simulink model "CurrentRegulationandFeedbackComponent"  (R2026a)
settings: Solver=FixedStepDiscrete
settings Model: DataDictionary=TractionEmotorSoftwareArchInterfaceData.sldd  Creator=dakaihu  LastModifiedBy=dakaihu

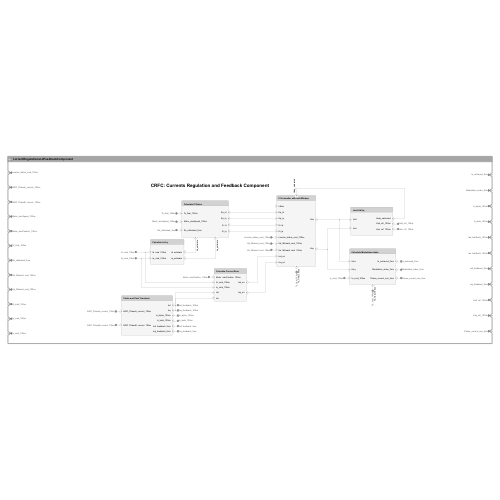
[thumbnail: Simulink's stored preview of the top-level diagram]
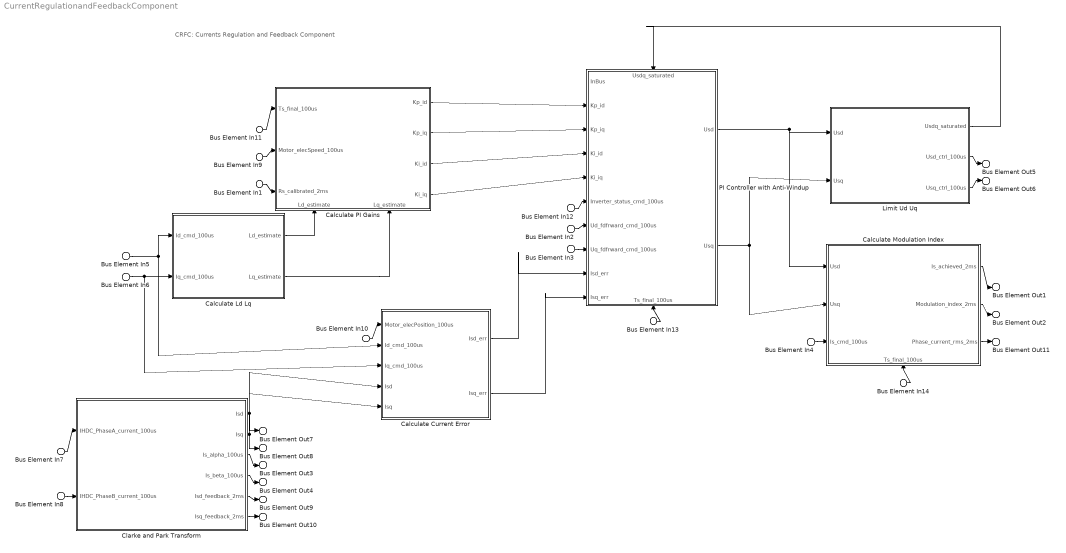
== system CurrentRegulationandFeedbackComponent ==
  note: CRFC: Currents Regulation and Feedback Component
  Bus Element In12 : Inport  PortName=Inverter_status_cmd_100us
  Bus Element In7 : Inport  Port=2  PortName=IHDC_PhaseA_current_100us
  Bus Element In8 : Inport  Port=3  PortName=IHDC_PhaseB_current_100us
  Bus Element In9 : Inport  Port=4  PortName=Motor_elecSpeed_100us
  Bus Element In10 : Inport  Port=5  PortName=Motor_elecPosition_100us
  Bus Element In11 : Inport  Port=6  PortName=Ts_final_100us
  Bus Element In13 : Inport  Port=6  PortName=Ts_final_100us
  Bus Element In14 : Inport  Port=6  PortName=Ts_final_100us
  Bus Element In1 : Inport  Port=7  PortName=Rs_calibrated_2ms
  Bus Element In2 : Inport  Port=8  PortName=Ud_fdfrward_cmd_100us
  Bus Element In3 : Inport  Port=9  PortName=Uq_fdfrward_cmd_100us
  Bus Element In5 : Inport  Port=10  PortName=Id_cmd_100us
  Bus Element In6 : Inport  Port=11  PortName=Iq_cmd_100us
  Bus Element In4 : Inport  Port=12  PortName=Is_cmd_100us
  "Calculate Current Error " : Subsystem
      settings: PortSchema="{\"entries\":[{\"content\":{\"headerSize\":26,\"margin\":15,\"minimumSpacing\":25,\"sides\":[{\"content\":{\"connectorIds\":[\"In1\",\"In2\",\"In3\",\"In4\",\"In5\"]},\"type\":\"ConnectorPlacement.EquallySpacedRectSide\",\"uuid\":\"48197cfa-225d-469b-bade-a4603c3ad603\"},{\"content\":{\"connectorIds\":[\"Out1\",\"Out2\"],\"side\":\"RIGHT\"},\"type\":\"ConnectorPlacement.EquallySpacedRectSide\",\"uuid\":\"66f990f6-adbc-4e6f-80ea-1c4f0b5a4b64\"},{\"content\":{\"connectorIds\":[],\"side\":\"TOP\"},\"type\":\"ConnectorPlacement.EquallySpacedRectSide\",\"uuid\":\"942001c3-a853-4b04-81e7-4a7a1fb8bb28\"}]},\"type\":\"ConnectorPlacement.EquallySpacedConnector\",\"uuid\":\"eed822cb-7078-4505-8d8e-0c793411ce34\"}],\"packageUris\":[\"http://schema.mathworks.com/mf0/Connector/R2020b\"],\"version\":\"1.0\"}"
  Calculate Ld Lq : Subsystem
      settings: PortSchema="{\"entries\":[{\"content\":{\"headerSize\":26,\"margin\":15,\"minimumSpacing\":25,\"sides\":[{\"content\":{\"connectorIds\":[\"In1\",\"In2\"]},\"type\":\"ConnectorPlacement.EquallySpacedRectSide\",\"uuid\":\"48197cfa-225d-469b-bade-a4603c3ad603\"},{\"content\":{\"connectorIds\":[\"Out1\",\"Out2\"],\"side\":\"RIGHT\"},\"type\":\"ConnectorPlacement.EquallySpacedRectSide\",\"uuid\":\"66f990f6-adbc-4e6f-80ea-1c4f0b5a4b64\"},{\"content\":{\"connectorIds\":[],\"side\":\"TOP\"},\"type\":\"ConnectorPlacement.EquallySpacedRectSide\",\"uuid\":\"942001c3-a853-4b04-81e7-4a7a1fb8bb28\"}]},\"type\":\"ConnectorPlacement.EquallySpacedConnector\",\"uuid\":\"eed822cb-7078-4505-8d8e-0c793411ce34\"}],\"packageUris\":[\"http://schema.mathworks.com/mf0/Connector/R2020b\"],\"version\":\"1.0\"}"
  Calculate Modulation Index : Subsystem
      settings: PortSchema="{\"entries\":[{\"content\":{\"headerSize\":26,\"margin\":15,\"minimumSpacing\":25,\"sides\":[{\"content\":{\"connectorIds\":[\"In2\",\"In3\",\"In4\"]},\"type\":\"ConnectorPlacement.EquallySpacedRectSide\",\"uuid\":\"48197cfa-225d-469b-bade-a4603c3ad603\"},{\"content\":{\"connectorIds\":[\"Out1\",\"Out2\",\"Out3\"],\"side\":\"RIGHT\"},\"type\":\"ConnectorPlacement.EquallySpacedRectSide\",\"uuid\":\"66f990f6-adbc-4e6f-80ea-1c4f0b5a4b64\"},{\"content\":{\"connectorIds\":[],\"side\":\"TOP\"},\"type\":\"ConnectorPlacement.EquallySpacedRectSide\",\"uuid\":\"942001c3-a853-4b04-81e7-4a7a1fb8bb28\"},{\"content\":{\"connectorIds\":[\"In1\"],\"side\":\"BOTTOM\"},\"type\":\"ConnectorPlacement.EquallySpacedRectSide\",\"uuid\":\"b02502b0-0db1-4dfc-a3e2-057df5b912de\"}]},\"type\":\"ConnectorPlacement.EquallySpacedConnector\",\"uuid\":\"eed822cb-7078-4505-8d8e-0c793411ce34\"}],\"packageUris\":[\"http://schema.mathworks.com/mf0/Connector/R2020b\"],\"version\":\"1.0\"}"
  Calculate PI Gains : Subsystem
      settings: PortSchema="{\"entries\":[{\"content\":{\"headerSize\":26,\"margin\":15,\"minimumSpacing\":25,\"sides\":[{\"content\":{\"connectorIds\":[\"In1\",\"In2\",\"In3\"]},\"type\":\"ConnectorPlacement.EquallySpacedRectSide\",\"uuid\":\"48197cfa-225d-469b-bade-a4603c3ad603\"},{\"content\":{\"connectorIds\":[\"Out1\",\"Out2\",\"Out4\",\"Out3\"],\"side\":\"RIGHT\"},\"type\":\"ConnectorPlacement.EquallySpacedRectSide\",\"uuid\":\"66f990f6-adbc-4e6f-80ea-1c4f0b5a4b64\"},{\"content\":{\"connectorIds\":[],\"side\":\"TOP\"},\"type\":\"ConnectorPlacement.EquallySpacedRectSide\",\"uuid\":\"942001c3-a853-4b04-81e7-4a7a1fb8bb28\"},{\"content\":{\"connectorIds\":[\"In4\",\"In5\"],\"side\":\"BOTTOM\"},\"type\":\"ConnectorPlacement.EquallySpacedRectSide\",\"uuid\":\"3d9d326e-8475-49e8-bdf1-4ba0dc1e2f42\"}]},\"type\":\"ConnectorPlacement.EquallySpacedConnector\",\"uuid\":\"eed822cb-7078-4505-8d8e-0c793411ce34\"}],\"packageUris\":[\"http://schema.mathworks.com/mf0/Connector/R2020b\"],\"version\":\"1.0\"}"
  Clarke and Park Transform : Subsystem
      settings: PortSchema="{\"entries\":[{\"content\":{\"headerSize\":26,\"margin\":15,\"minimumSpacing\":25,\"sides\":[{\"content\":{\"connectorIds\":[\"In1\",\"In2\"]},\"type\":\"ConnectorPlacement.EquallySpacedRectSide\",\"uuid\":\"48197cfa-225d-469b-bade-a4603c3ad603\"},{\"content\":{\"connectorIds\":[\"Out1\",\"Out2\",\"Out3\",\"Out4\",\"Out5\",\"Out6\"],\"side\":\"RIGHT\"},\"type\":\"ConnectorPlacement.EquallySpacedRectSide\",\"uuid\":\"66f990f6-adbc-4e6f-80ea-1c4f0b5a4b64\"},{\"content\":{\"connectorIds\":[],\"side\":\"TOP\"},\"type\":\"ConnectorPlacement.EquallySpacedRectSide\",\"uuid\":\"942001c3-a853-4b04-81e7-4a7a1fb8bb28\"}]},\"type\":\"ConnectorPlacement.EquallySpacedConnector\",\"uuid\":\"eed822cb-7078-4505-8d8e-0c793411ce34\"}],\"packageUris\":[\"http://schema.mathworks.com/mf0/Connector/R2020b\"],\"version\":\"1.0\"}"
  Limit Ud Uq : Subsystem
      settings: PortSchema="{\"entries\":[{\"content\":{\"headerSize\":26,\"margin\":15,\"minimumSpacing\":25,\"sides\":[{\"content\":{\"connectorIds\":[\"In1\",\"In2\"]},\"type\":\"ConnectorPlacement.EquallySpacedRectSide\",\"uuid\":\"48197cfa-225d-469b-bade-a4603c3ad603\"},{\"content\":{\"connectorIds\":[\"Out1\",\"Out2\",\"Out3\"],\"side\":\"RIGHT\"},\"type\":\"ConnectorPlacement.EquallySpacedRectSide\",\"uuid\":\"66f990f6-adbc-4e6f-80ea-1c4f0b5a4b64\"},{\"content\":{\"connectorIds\":[],\"side\":\"TOP\"},\"type\":\"ConnectorPlacement.EquallySpacedRectSide\",\"uuid\":\"942001c3-a853-4b04-81e7-4a7a1fb8bb28\"}]},\"type\":\"ConnectorPlacement.EquallySpacedConnector\",\"uuid\":\"eed822cb-7078-4505-8d8e-0c793411ce34\"}],\"packageUris\":[\"http://schema.mathworks.com/mf0/Connector/R2020b\"],\"version\":\"1.0\"}"
  PI Controller with Anti-Windup : Subsystem
      settings: PortSchema="{\"entries\":[{\"content\":{\"headerSize\":26,\"margin\":15,\"minimumSpacing\":25,\"sides\":[{\"content\":{\"connectorIds\":[\"In2\",\"In5\",\"In6\",\"In7\",\"In8\",\"In4\",\"In9\",\"In10\",\"In11\",\"In12\"]},\"type\":\"ConnectorPlacement.EquallySpacedRectSide\",\"uuid\":\"48197cfa-225d-469b-bade-a4603c3ad603\"},{\"content\":{\"connectorIds\":[\"Out1\",\"Out2\"],\"side\":\"RIGHT\"},\"type\":\"ConnectorPlacement.EquallySpacedRectSide\",\"uuid\":\"66f990f6-adbc-4e6f-80ea-1c4f0b5a4b64\"},{\"content\":{\"connectorIds\":[\"In3\"],\"side\":\"TOP\"},\"type\":\"ConnectorPlacement.EquallySpacedRectSide\",\"uuid\":\"942001c3-a853-4b04-81e7-4a7a1fb8bb28\"},{\"content\":{\"connectorIds\":[\"In1\"],\"side\":\"BOTTOM\"},\"type\":\"ConnectorPlacement.EquallySpacedRectSide\",\"uuid\":\"cc117984-18a2-4a20-b6dc-41212c4c98a4\"}]},\"type\":\"ConnectorPlacement.EquallySpacedConnector\",\"uuid\":\"eed822cb-7078-4505-8d8e-0c793411ce34\"}],\"packageUris\":[\"http://schema.mathworks.com/mf0/Connector/R2020b\"],\"version\":\"1.0\"}"
  Bus Element Out1 : Outport  PortName=Is_achieved_2ms
  Bus Element Out2 : Outport  Port=2  PortName=Modulation_index_2ms
  Bus Element Out3 : Outport  Port=3  PortName=Is_alpha_100us
  Bus Element Out4 : Outport  Port=4  PortName=Is_beta_100us
  Bus Element Out7 : Outport  Port=5  PortName=Isd_feedback_100us
  Bus Element Out8 : Outport  Port=6  PortName=Isq_feedback_100us
  Bus Element Out9 : Outport  Port=7  PortName=Isd_feedback_2ms
  Bus Element Out10 : Outport  Port=8  PortName=Isq_feedback_2ms
  Bus Element Out5 : Outport  Port=9  PortName=Usd_ctrl_100us
  Bus Element Out6 : Outport  Port=10  PortName=Usq_ctrl_100us
  Bus Element Out11 : Outport  Port=11  PortName=Phase_current_rms_2ms
  wires:
  Bus Element In5/1 -> "Calculate Current Error "/2(Id_cmd_100us), Calculate Ld Lq/1(Id_cmd_100us)
  Bus Element In6/1 -> "Calculate Current Error "/3(Iq_cmd_100us), Calculate Ld Lq/2(Iq_cmd_100us)
  Calculate Ld Lq/1(Ld_estimate) -> Calculate PI Gains/4(Ld_estimate)
  Calculate Ld Lq/2(Lq_estimate) -> Calculate PI Gains/5(Lq_estimate)
  Bus Element In11/1 -> Calculate PI Gains/1(Ts_final_100us)
  Bus Element In9/1 -> Calculate PI Gains/2(Motor_elecSpeed_100us)
  Bus Element In1/1 -> Calculate PI Gains/3(Rs_calibrated_2ms)
  Calculate PI Gains/1(Kp_id) -> PI Controller with Anti-Windup/5(Kp_id)
  Calculate PI Gains/2(Kp_iq) -> PI Controller with Anti-Windup/6(Kp_iq)
  Calculate PI Gains/4(Ki_id) -> PI Controller with Anti-Windup/7(Ki_id)
  Calculate PI Gains/3(Ki_iq) -> PI Controller with Anti-Windup/8(Ki_iq)
  Bus Element In2/1 -> PI Controller with Anti-Windup/9(Ud_fdfrward_cmd_100us)
  Bus Element In3/1 -> PI Controller with Anti-Windup/10(Uq_fdfrward_cmd_100us)
  Bus Element In12/1 -> PI Controller with Anti-Windup/4(Inverter_status_cmd_100us)
  "Calculate Current Error "/1(Isd_err) -> PI Controller with Anti-Windup/11(Isd_err)
  "Calculate Current Error "/2(Isq_err) -> PI Controller with Anti-Windup/12(Isq_err)
  Bus Element In7/1 -> Clarke and Park Transform/1(IHDC_PhaseA_current_100us)
  Bus Element In8/1 -> Clarke and Park Transform/2(IHDC_PhaseB_current_100us)
  Clarke and Park Transform/3(Is_alpha_100us) -> Bus Element Out3/1
  Clarke and Park Transform/4(Is_beta_100us) -> Bus Element Out4/1
  Bus Element In10/1 -> "Calculate Current Error "/1(Motor_elecPosition_100us)
  PI Controller with Anti-Windup/2(Usq) -> Limit Ud Uq/2(Usq), Calculate Modulation Index/3(Usq)
  Limit Ud Uq/1(Usdq_saturated) -> PI Controller with Anti-Windup/3(Usdq_saturated)
  Bus Element In4/1 -> Calculate Modulation Index/4(Is_cmd_100us)
  Bus Element In13/1 -> PI Controller with Anti-Windup/1(Ts_final_100us)
  Bus Element In14/1 -> Calculate Modulation Index/1(Ts_final_100us)
  Clarke and Park Transform/1(Isd) -> "Calculate Current Error "/4(Isd), Bus Element Out7/1
  Clarke and Park Transform/2(Isq) -> "Calculate Current Error "/5(Isq), Bus Element Out8/1
  Clarke and Park Transform/5(Isd_feedback_2ms) -> Bus Element Out9/1
  Clarke and Park Transform/6(Isq_feedback_2ms) -> Bus Element Out10/1
  Calculate Modulation Index/1(Is_achieved_2ms) -> Bus Element Out1/1
  Calculate Modulation Index/2(Modulation_index_2ms) -> Bus Element Out2/1
  PI Controller with Anti-Windup/1(Usd) -> Limit Ud Uq/1(Usd), Calculate Modulation Index/2(Usd)
  Limit Ud Uq/2(Usd_ctrl_100us) -> Bus Element Out5/1
  Limit Ud Uq/3(Usq_ctrl_100us) -> Bus Element Out6/1
  Calculate Modulation Index/3(Phase_current_rms_2ms) -> Bus Element Out11/1

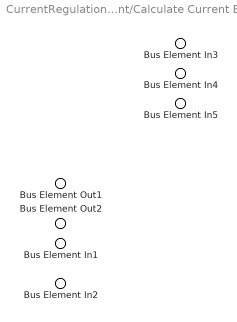
== system CurrentRegulationandFeedbackComponent/Calculate Current Error  ==
  Bus Element In5 : Inport  PortName=Motor_elecPosition_100us
  Bus Element In3 : Inport  Port=2  PortName=Id_cmd_100us
  Bus Element In4 : Inport  Port=3  PortName=Iq_cmd_100us
  Bus Element In1 : Inport  Port=4  PortName=Isd
  Bus Element In2 : Inport  Port=5  PortName=Isq
  Bus Element Out1 : Outport  PortName=Isd_err
  Bus Element Out2 : Outport  Port=2  PortName=Isq_err

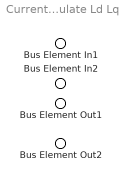
== system CurrentRegulationandFeedbackComponent/Calculate Ld Lq ==
  Bus Element In1 : Inport  PortName=Id_cmd_100us
  Bus Element In2 : Inport  Port=2  PortName=Iq_cmd_100us
  Bus Element Out1 : Outport  PortName=Ld_estimate
  Bus Element Out2 : Outport  Port=2  PortName=Lq_estimate

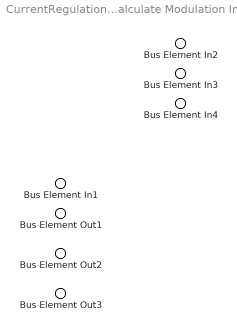
== system CurrentRegulationandFeedbackComponent/Calculate Modulation Index ==
  Bus Element In4 : Inport  PortName=Ts_final_100us
  Bus Element In3 : Inport  Port=2  PortName=Usd
  Bus Element In2 : Inport  Port=3  PortName=Usq
  Bus Element In1 : Inport  Port=4  PortName=Is_cmd_100us
  Bus Element Out1 : Outport  PortName=Is_achieved_2ms
  Bus Element Out2 : Outport  Port=2  PortName=Modulation_index_2ms
  Bus Element Out3 : Outport  Port=3  PortName=Phase_current_rms_2ms

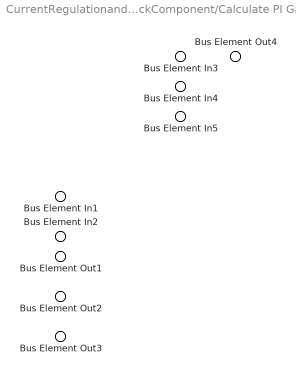
== system CurrentRegulationandFeedbackComponent/Calculate PI Gains ==
  Bus Element In3 : Inport  PortName=Ts_final_100us
  Bus Element In4 : Inport  Port=2  PortName=Motor_elecSpeed_100us
  Bus Element In5 : Inport  Port=3  PortName=Rs_calibrated_2ms
  Bus Element In1 : Inport  Port=4  PortName=Ld_estimate
  Bus Element In2 : Inport  Port=5  PortName=Lq_estimate
  Bus Element Out1 : Outport  PortName=Kp_id
  Bus Element Out2 : Outport  Port=2  PortName=Kp_iq
  Bus Element Out4 : Outport  Port=3  PortName=Ki_iq
  Bus Element Out3 : Outport  Port=4  PortName=Ki_id

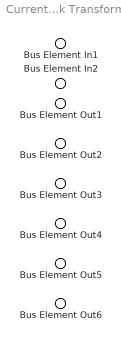
== system CurrentRegulationandFeedbackComponent/Clarke and Park Transform ==
  Bus Element In1 : Inport  PortName=IHDC_PhaseA_current_100us
  Bus Element In2 : Inport  Port=2  PortName=IHDC_PhaseB_current_100us
  Bus Element Out1 : Outport  PortName=Isd
  Bus Element Out2 : Outport  Port=2  PortName=Isq
  Bus Element Out3 : Outport  Port=3  PortName=Is_alpha_100us
  Bus Element Out4 : Outport  Port=4  PortName=Is_beta_100us
  Bus Element Out5 : Outport  Port=5  PortName=Isd_feedback_2ms
  Bus Element Out6 : Outport  Port=6  PortName=Isq_feedback_2ms

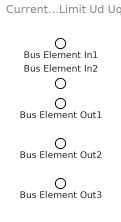
== system CurrentRegulationandFeedbackComponent/Limit Ud Uq ==
  Bus Element In1 : Inport  PortName=Usd
  Bus Element In2 : Inport  Port=2  PortName=Usq
  Bus Element Out1 : Outport  PortName=Usdq_saturated
  Bus Element Out2 : Outport  Port=2  PortName=Usd_ctrl_100us
  Bus Element Out3 : Outport  Port=3  PortName=Usq_ctrl_100us

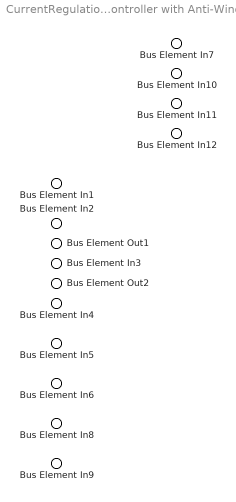
== system CurrentRegulationandFeedbackComponent/PI Controller with Anti-Windup ==
  Bus Element In12 : Inport  PortName=Ts_final_100us
  Bus Element In11 : Inport  Port=2  PortName=InBus
  Bus Element In10 : Inport  Port=3  PortName=Usdq_saturated
  Bus Element In7 : Inport  Port=4  PortName=Inverter_status_cmd_100us
  Bus Element In1 : Inport  Port=5  PortName=Kp_id
  Bus Element In2 : Inport  Port=6  PortName=Kp_iq
  Bus Element In3 : Inport  Port=7  PortName=Ki_id
  Bus Element In4 : Inport  Port=8  PortName=Ki_iq
  Bus Element In5 : Inport  Port=9  PortName=Ud_fdfrward_cmd_100us
  Bus Element In6 : Inport  Port=10  PortName=Uq_fdfrward_cmd_100us
  Bus Element In8 : Inport  Port=11  PortName=Isd_err
  Bus Element In9 : Inport  Port=12  PortName=Isq_err
  Bus Element Out1 : Outport  PortName=Usd
  Bus Element Out2 : Outport  Port=2  PortName=Usq
